simulink model "VVI_state"  (R2020a)
settings: Solver=FixedStepAuto  StartTime=0.0  StopTime=10.0  FixedStep=1e-3  RelTol=1e-3  EnableMultiTasking=on
undefined symbols (not defined in the file): D1, D10, D11, D12, D13, D2, D3, D4, D5, D7, D8, D9, PTA0, PTA1, PTA2, PTB23, PTB9, PTC17, PTC3, PTC4, PTD0, PTD1, PTD2, PTD3
libraries: frdmk64flib x16
settings Model: ExtModeTrigDuration=5  Creator=ahmed  LastModifiedBy=Faisal
settings OptimizationCC: EnhancedBackFolding=on  PassReuseOutputArgsAs=Individual arguments  ZeroExternalMemoryAtStartup=off  ZeroInternalMemoryAtStartup=off  MaxStackSize=64  OptimizeBlockOrder=speed  DifferentSizesBufferReuse=on  OptimizationCustomize=off  EfficientTunableParamExpr=on
settings DebuggingCC: ParameterTunabilityLossMsg=error
settings HardwareCC: ProdBitPerPointer=32  ProdBitPerSizeT=32  ProdBitPerPtrDiffT=32  ProdLargestAtomicInteger=Long  ProdLargestAtomicFloat=Double  ProdWordSize=32  ProdHWDeviceType=ARM Compatible->ARM Cortex
settings SFSimCC: MATLABDynamicMemAlloc=off
settings RTWCC: SystemTargetFile=ert.tlc  HardwareBoard=NXP FRDM-K64F  TemplateMakefile=ert_default_tmf  Toolchain=GNU Tools for ARM Embedded Processors
settings CodeAppCC: ForceParamTrailComments=on  IgnoreCustomStorageClasses=off  OperatorAnnotations=on  SimulinkDataObjDesc=on  SFDataObjDesc=on  InsertBlockDesc=on

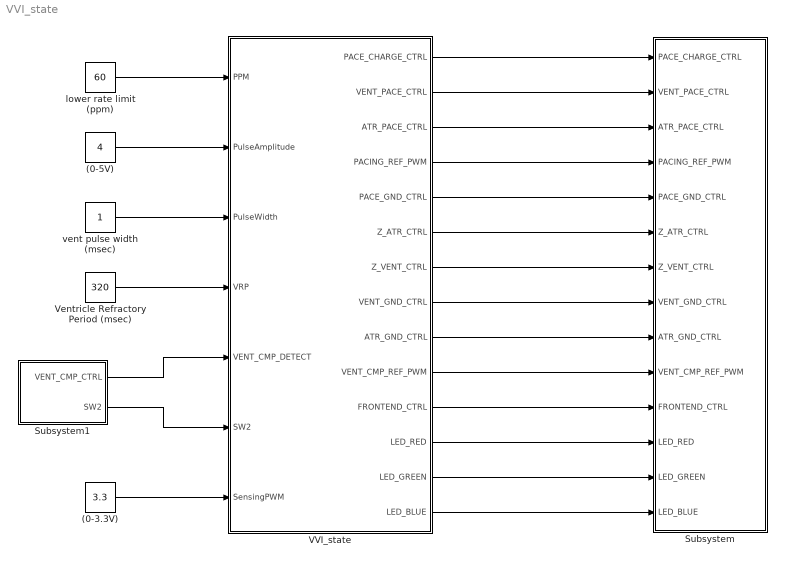
== system VVI_state ==
  (0-3.3V) : Constant  Value=3.3
  (0-5V) : Constant  Value=4
  Subsystem : Subsystem
  Subsystem1 : Subsystem
  VVI_state : Stateflow chart  TreatAsAtomicUnit=on
  Ventricle Refractory Period (msec) : Constant  Value=320
  lower rate limit (ppm) : Constant  Value=60
  vent pulse width (msec) : Constant
  wires:
  lower rate limit (ppm)/1 -> VVI_state/1(PPM)
  (0-5V)/1 -> VVI_state/2(PulseAmplitude)
  vent pulse width (msec)/1 -> VVI_state/3(PulseWidth)
  Ventricle Refractory Period (msec)/1 -> VVI_state/4(VRP)
  (0-3.3V)/1 -> VVI_state/7(SensingPWM)
  VVI_state/1(PACE_CHARGE_CTRL) -> Subsystem/1(PACE_CHARGE_CTRL)
  VVI_state/2(VENT_PACE_CTRL) -> Subsystem/2(VENT_PACE_CTRL)
  VVI_state/3(ATR_PACE_CTRL) -> Subsystem/3(ATR_PACE_CTRL)
  VVI_state/4(PACING_REF_PWM) -> Subsystem/4(PACING_REF_PWM)
  VVI_state/5(PACE_GND_CTRL) -> Subsystem/5(PACE_GND_CTRL)
  VVI_state/6(Z_ATR_CTRL) -> Subsystem/6(Z_ATR_CTRL)
  VVI_state/7(Z_VENT_CTRL) -> Subsystem/7(Z_VENT_CTRL)
  VVI_state/8(VENT_GND_CTRL) -> Subsystem/8(VENT_GND_CTRL)
  VVI_state/9(ATR_GND_CTRL) -> Subsystem/9(ATR_GND_CTRL)
  VVI_state/10(VENT_CMP_REF_PWM) -> Subsystem/10(VENT_CMP_REF_PWM)
  VVI_state/11(FRONTEND_CTRL) -> Subsystem/11(FRONTEND_CTRL)
  VVI_state/12(LED_RED) -> Subsystem/12(LED_RED)
  VVI_state/13(LED_GREEN) -> Subsystem/13(LED_GREEN)
  VVI_state/14(LED_BLUE) -> Subsystem/14(LED_BLUE)
  Subsystem1/1(VENT_CMP_CTRL) -> VVI_state/5(VENT_CMP_DETECT)
  Subsystem1/2(SW2) -> VVI_state/6(SW2)

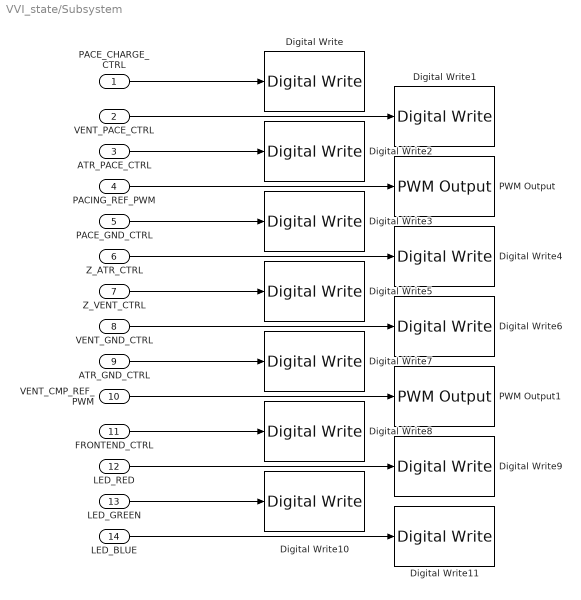
== system VVI_state/Subsystem ==
  PACE_CHARGE_CTRL : Inport
  VENT_PACE_CTRL : Inport  Port=2
  ATR_PACE_CTRL : Inport  Port=3
  PACING_REF_PWM : Inport  Port=4
  PACE_GND_CTRL : Inport  Port=5
  Z_ATR_CTRL : Inport  Port=6
  Z_VENT_CTRL : Inport  Port=7
  VENT_GND_CTRL : Inport  Port=8
  ATR_GND_CTRL : Inport  Port=9
  VENT_CMP_REF_PWM : Inport  Port=10
  FRONTEND_CTRL : Inport  Port=11
  LED_RED : Inport  Port=12
  LED_GREEN : Inport  Port=13
  LED_BLUE : Inport  Port=14
  Digital Write : frdmk64flib/Digital Write  Whichpin=PTB9 (D2)
  Digital Write1 : frdmk64flib/Digital Write  Whichpin=PTC4 (D9)
  Digital Write10 : frdmk64flib/Digital Write  Whichpin=GREEN_LED
  Digital Write11 : frdmk64flib/Digital Write  Whichpin=BLUE_LED
  Digital Write2 : frdmk64flib/Digital Write  Whichpin=PTA0 (D8)
  Digital Write3 : frdmk64flib/Digital Write  Whichpin=PTD0 (D10)
  Digital Write4 : frdmk64flib/Digital Write  Whichpin=PTB23 (D4)
  Digital Write5 : frdmk64flib/Digital Write  Whichpin=PTC3 (D7)
  Digital Write6 : frdmk64flib/Digital Write  Whichpin=PTD3 (D12)
  Digital Write7 : frdmk64flib/Digital Write  Whichpin=PTD2 (D11)
  Digital Write8 : frdmk64flib/Digital Write  Whichpin=PTD1 (D13)
  Digital Write9 : frdmk64flib/Digital Write  Whichpin=RED_LED
  PWM Output : frdmk64flib/PWM Output  Whichpin=PTA2 (D5)  InitialFrequency=2000  InitialDutyCycle=0
  PWM Output1 : frdmk64flib/PWM Output  Whichpin=PTA1 (D3)  InitialFrequency=2000  InitialDutyCycle=0
  wires:
  VENT_GND_CTRL/1 -> Digital Write6/1
  VENT_CMP_REF_PWM/1 -> PWM Output1/1
  PACE_CHARGE_CTRL/1 -> Digital Write/1
  FRONTEND_CTRL/1 -> Digital Write8/1
  ATR_GND_CTRL/1 -> Digital Write7/1
  PACING_REF_PWM/1 -> PWM Output/1
  VENT_PACE_CTRL/1 -> Digital Write1/1
  LED_GREEN/1 -> Digital Write10/1
  LED_RED/1 -> Digital Write9/1
  ATR_PACE_CTRL/1 -> Digital Write2/1
  PACE_GND_CTRL/1 -> Digital Write3/1
  Z_VENT_CTRL/1 -> Digital Write5/1
  LED_BLUE/1 -> Digital Write11/1
  Z_ATR_CTRL/1 -> Digital Write4/1

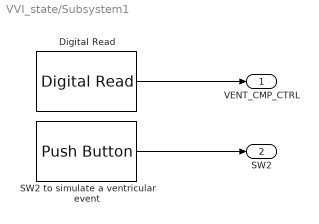
== system VVI_state/Subsystem1 ==
  Digital Read : frdmk64flib/Digital Read  Whichpin=PTC17 (D1)  SampleTime=-1
  SW2 to simulate a ventricular event : frdmk64flib/Push Button  Whichswitch=SW2  SampleTime1=-1
  VENT_CMP_CTRL : Outport
  SW2 : Outport  Port=2
  wires:
  SW2 to simulate a ventricular event/1 -> SW2/1
  Digital Read/1 -> VENT_CMP_CTRL/1

== stateflow chart VVI_state/VVI_state ==
  state Charging_C22
    entry:
    %Charging C22
    PACE_CHARGE_CTRL=true;
    VENT_PACE_CTRL=false;
    ATR_PACE_CTRL=false;
    PACING_REF_PWM=20*PulseAmplitude;
    %Discharging C21
    PACE_GND_CTRL=true;
    Z_ATR_CTRL=false;
    Z_VENT_CTRL=false;
    ATR_PACE_CTRL=false;
    VENT_GND_CTRL=true;
    ATR_GND_CTRL=false;
    VENT_CMP_REF_PWM=30*SensingPWM;
    FRONTEND_CTRL=true;
    %Turn Red on
    LED_RED=true;
    LED_GREEN=false;
    LED_BLUE=false;
  state Sense_and_Inhibit
    entry:
    PACING_REF_PWM = 20*PulseAmplitude;
    PACE_CHARGE_CTRL=true;
    %Discharging C21
    PACE_GND_CTRL=true;
    VENT_GND_CTRL=true;
    %Turn Blue ON
    LED_GREEN=false;
    LED_BLUE=true;
    LED_RED=false;
  state Pacing_Ventricle
    entry:
    PACE_CHARGE_CTRL=false;
    PACE_GND_CTRL=true;
    ATR_PACE_CTRL=false;
    ATR_GND_CTRL=false;
    VENT_PACE_CTRL=true;
    VENT_GND_CTRL=false;
    Z_ATR_CTRL=false;
    Z_VENT_CTRL=false;
    %Turn Green on
    LED_GREEN=true;
    LED_RED=false;
    LED_BLUE=false;
  (default) -> Charging_C22
  Charging_C22 -> Sense_and_Inhibit [order 1] : [VENT_CMP_DETECT==true | SW2==true]
  Pacing_Ventricle -> Sense_and_Inhibit : after(PulseWidth,msec)
  Sense_and_Inhibit -> Charging_C22 : after(VRP,msec)
  Charging_C22 -> Pacing_Ventricle [order 2] : after((60000/PPM)-VRP-PulseWidth,msec)[VENT_CMP_DETECT==false & SW2==false]
  data: PACE_CHARGE_CTRL output boolean; VENT_PACE_CTRL output boolean; ATR_PACE_CTRL output boolean; PACING_REF_PWM output double; PACE_GND_CTRL output boolean; Z_ATR_CTRL output boolean; Z_VENT_CTRL output boolean; VENT_GND_CTRL output boolean; ATR_GND_CTRL output boolean; VENT_CMP_REF_PWM output double; FRONTEND_CTRL output; LED_RED output; LED_GREEN output; LED_BLUE output; PPM input double; PulseAmplitude input double; PulseWidth input double; VRP input double; VENT_CMP_DETECT input boolean; SW2 input boolean; SensingPWM input double
